simulink model "LinearModel_RudderActuator"  (R2012b)
settings: Solver=ode23s  StartTime=0.0  StopTime=5  FixedStep=1e-4  RelTol=1e-3
values from neighbouring files (symbols this model uses):
  StateControl =     [StateControl.mat]
undefined symbols (not defined in the file or in its folder): C, EHSV_Step, L0, Max_Cmd, Min_Cmd, R, Rate_Limit, sys_act, T_ES, Theta0, X0
settings Model: Creator=HERIC  LastModifiedBy=HBALLEST

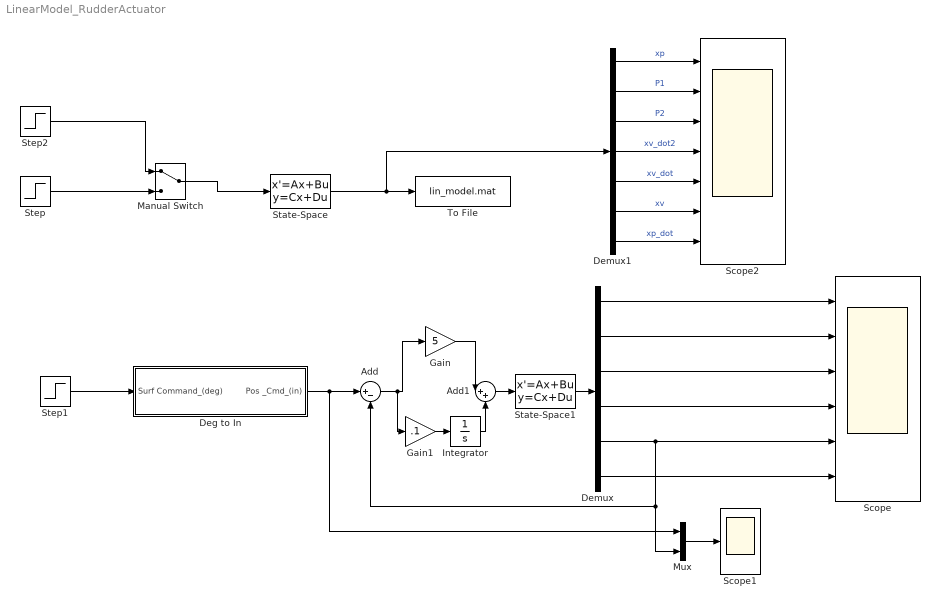
== system LinearModel_RudderActuator ==
  Add : Sum  Inputs=|+-
  Add1 : Sum  Inputs=|++
  Deg to In : Subsystem
  Demux : Demux  Outputs=6
  Demux1 : Demux  Outputs=7
  Gain : Gain  Gain=5
  Gain1 : Gain  Gain=.1
  Integrator : Integrator
  Manual Switch : ManualSwitch
  Mux : Mux  Inputs=2
  Scope : Scope  NumInputPorts=6
      settings: YMin=-5~-5~-5~-5~-5~-5  YMax=5~5~5~5~5~5
  Scope1 : Scope
      settings: TimeRange=5  YMin=-0.002  YMax=0.016
  Scope2 : Scope  NumInputPorts=7
      settings: TimeRange=1.515675675675676  YMin=-5.909099753670425e-26~-400000~0~-6.086956521739157e-06~-1.154319942386694e-20~-5e-06~-1e-09  YMax=0.06710526315789475~200000~300000~3.391304347826084e-05~0.04~5e-06~2.000000000000001e-09  SaveName=ScopeData2
  State-Space : StateSpace  A=StateControl.A  B=StateControl.B  C=eye(7)  D=zeros(7,1)  X0=StateControl.X0
  State-Space1 : StateSpace  A=sys_act.A  B=sys_act.B  C=eye(7)  D=zeros(7,1)  X0=X0
  Step : Step  Time=EHSV_Step.time  Before=EHSV_Step.initial  After=EHSV_Step.final
  Step1 : Step  Time=.5  After=30  SampleTime=1e-3
  Step2 : Step  Time=0.5  After=8
  To File : ToFile  Filename=lin_model.mat  MatrixName=states_lin  SaveFormat=Timeseries
  wires:
  Step/1 -> Manual Switch/2
  State-Space/1 -> Demux1/1, To File/1
  State-Space1/1 -> Demux/1
  Demux/1 -> Scope/1
  Demux/2 -> Scope/2
  Demux/3 -> Scope/3
  Demux/4 -> Scope/4
  Demux/5 -> Add/2, Mux/2, Scope/5
  Demux/6 -> Scope/6
  Step1/1 -> Deg to In/1(Surf Command_(deg))
  Deg to In/1(Pos _Cmd_(in)) -> Add/1, Mux/1
  Add/1 -> Gain1/1, Gain/1
  Mux/1 -> Scope1/1
  Gain/1 -> Add1/1
  Integrator/1 -> Add1/2
  Add1/1 -> State-Space1/1
  Gain1/1 -> Integrator/1
  Demux1/7 -> Scope2/7  "xp_dot"
  Demux1/4 -> Scope2/4  "xv_dot2"
  Demux1/5 -> Scope2/5  "xv_dot"
  Demux1/2 -> Scope2/2  "P1"
  Demux1/1 -> Scope2/1  "xp"
  Demux1/3 -> Scope2/3  "P2"
  Manual Switch/1 -> State-Space/1
  Step2/1 -> Manual Switch/1
  Demux1/6 -> Scope2/6  "xv"

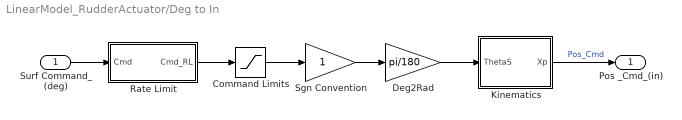
== system LinearModel_RudderActuator/Deg to In ==
  Surf Command_(deg) : Inport
  Command Limits : Saturate  UpperLimit=Max_Cmd  LowerLimit=Min_Cmd
  Deg2Rad : Gain  Gain=pi/180  SampleTime=T_ES  SaturateOnIntegerOverflow=on  OutDataTypeStr=Inherit: Same as input  ParamDataTypeStr=Inherit: Same as input
  Kinematics : Subsystem
  Rate Limit : Subsystem
  Sgn Convention : Gain  SampleTime=T_ES  SaturateOnIntegerOverflow=on  OutDataTypeStr=Inherit: Same as input  ParamDataTypeStr=Inherit: Same as input
  Pos _Cmd_(in) : Outport
  wires:
  Sgn Convention/1 -> Deg2Rad/1
  Rate Limit/1(Cmd_RL) -> Command Limits/1
  Surf Command_(deg)/1 -> Rate Limit/1(Cmd)
  Command Limits/1 -> Sgn Convention/1
  Kinematics/1(Xp) -> Pos _Cmd_(in)/1  "Pos_Cmd"
  Deg2Rad/1 -> Kinematics/1(ThetaS)

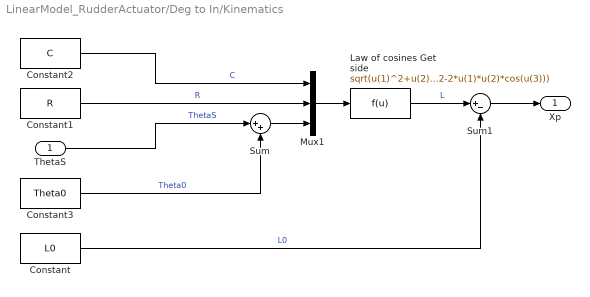
== system LinearModel_RudderActuator/Deg to In/Kinematics ==
  ThetaS : Inport
  Constant : Constant  Value=L0
  Constant1 : Constant  Value=R
  Constant2 : Constant  Value=C
  Constant3 : Constant  Value=Theta0
  Law of cosines Get side : Fcn  Expr=sqrt(u(1)^2+u(2)^2-2*u(1)*u(2)*cos(u(3)))  SampleTime=T_ES
  Mux1 : Mux  Inputs=3
  Sum : Sum  Inputs=|++  SampleTime=T_ES
  Sum1 : Sum  Inputs=|+-  SampleTime=T_ES
  Xp : Outport
  wires:
  Constant2/1 -> Mux1/1  "C"
  Constant1/1 -> Mux1/2  "R"
  Mux1/1 -> Law of cosines Get side/1
  ThetaS/1 -> Sum/1  "ThetaS"
  Sum/1 -> Mux1/3
  Law of cosines Get side/1 -> Sum1/1  "L"
  Constant/1 -> Sum1/2  "L0"
  Sum1/1 -> Xp/1
  Constant3/1 -> Sum/2  "Theta0"

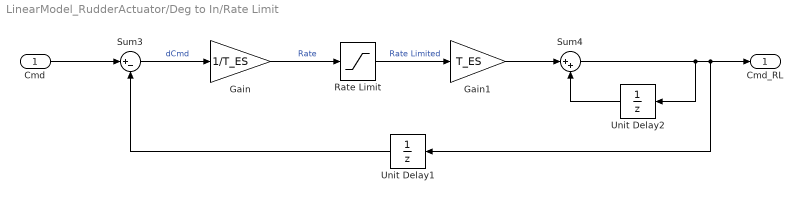
== system LinearModel_RudderActuator/Deg to In/Rate Limit ==
  Cmd : Inport
  Gain : Gain  Gain=1/T_ES
  Gain1 : Gain  Gain=T_ES
  Rate Limit : Saturate  UpperLimit=Rate_Limit  LowerLimit=-Rate_Limit
  Sum3 : Sum  Inputs=|+-  SaturateOnIntegerOverflow=on  InputSameDT=on  OutDataTypeStr=Inherit: Same as first input
  Sum4 : Sum  Inputs=|++  SaturateOnIntegerOverflow=on  InputSameDT=on  OutDataTypeStr=Inherit: Same as first input
  Unit Delay1 : UnitDelay  SampleTime=-1
  Unit Delay2 : UnitDelay  SampleTime=-1
  Cmd_RL : Outport
  wires:
  Cmd/1 -> Sum3/1
  Unit Delay1/1 -> Sum3/2
  Sum3/1 -> Gain/1  "dCmd"
  Gain/1 -> Rate Limit/1  "Rate"
  Rate Limit/1 -> Gain1/1  "Rate Limited"
  Unit Delay2/1 -> Sum4/2
  Sum4/1 -> Unit Delay2/1, Cmd_RL/1, Unit Delay1/1
  Gain1/1 -> Sum4/1
